simulink model "SAME5xPIM_MCLV2_MotorControl"  (R2020b)
settings: Solver=FixedStepDiscrete  StartTime=0.0  StopTime=10.0  FixedStep=0.0001  RelTol=1e-3  EnableMultiTasking=on
InitFcn:
  | % DC Voltage
  | VDC = 24;
  | 
  | % Intersective PMW
  | Vmax = VDC/2;
  | Imax = 4;
  | 
  | Ts = 1e-4;
  | 
  | 
  | % pole paires
  | p = 4;
  | 
  | % QEI
  | lines = 4*1000;
  | eleclines = lines/p;
  | inveleclines = 1/eleclines
  | gainQEIspeed = 2*pi/Ts/lines
  | 
  | % Electrical parameters
  | R=0.656; L=0.35e-3; Phif=0.0066;
  | % Mechanical parameters
  | F=1.e-05; J=1e-05; C0 = 0.01;%10;%1;
undefined symbols (not defined in the file or in its folder): ADC0, AIN0, DiscIntNeverNeededParam, PA02, PA03, PA08, PA09, PA10, PA11, PA12, PA13, PA16, PA17, PA18, pad0, pad1, pad2, pad3, PB08, PC16, PC17, PC18, Pin, SAME54P20A, TQFP128, VREFA, wo0, wo1, wo2, wo4, wo5, wo6
libraries: simulink x14, MCHP_Blockset x12, dsparch4 x1
(part 2 of 2)

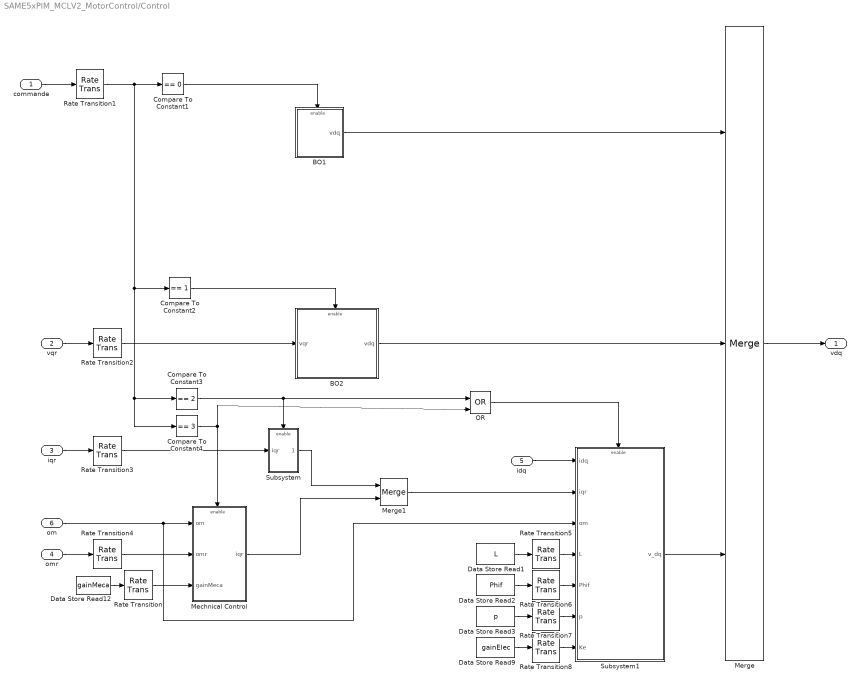
== system SAME5xPIM_MCLV2_MotorControl/Control ==
  commande : Inport
  vqr : Inport  Port=2
  iqr : Inport  Port=3
  omr : Inport  Port=4
  idq : Inport  Port=5
  om : Inport  Port=6
  BO1 : Subsystem
  BO2 : Subsystem
  Compare To Constant1 : simulink/Logic and Bit Operations/Compare To Constant  relop===  const=0  OutDataTypeStr=boolean
  Compare To Constant2 : simulink/Logic and Bit Operations/Compare To Constant  relop===  const=1  OutDataTypeStr=boolean
  Compare To Constant3 : simulink/Logic and Bit Operations/Compare To Constant  relop===  const=2  OutDataTypeStr=boolean
  Compare To Constant4 : simulink/Logic and Bit Operations/Compare To Constant  relop===  const=3  OutDataTypeStr=boolean
  Data Store Read1 : DataStoreRead  DataStoreName=L  SampleTime=1
  Data Store Read12 : DataStoreRead  DataStoreName=gainMeca  SampleTime=1
  Data Store Read2 : DataStoreRead  DataStoreName=Phif  SampleTime=1
  Data Store Read3 : DataStoreRead  DataStoreName=p  SampleTime=1
  Data Store Read9 : DataStoreRead  DataStoreName=gainElec  SampleTime=1
  Mechnical Control : Subsystem
  Merge : Merge  Inputs=3
  Merge1 : Merge
  OR : Logic  Operator=OR  IconShape=distinctive  AllPortsSameDT=off  OutDataTypeStr=boolean
  Rate Transition{,1..8} (9 alike) : RateTransition
  Subsystem : Subsystem
  Subsystem1 : Subsystem
  vdq : Outport  VectorParamsAs1DForOutWhenUnconnected=off
  wires:
  Rate Transition8/1 -> Subsystem1/7(Ke)
  Rate Transition7/1 -> Subsystem1/6(p)
  Rate Transition6/1 -> Subsystem1/5(Phif)
  Rate Transition5/1 -> Subsystem1/4(L)
  Rate Transition/1 -> Mechnical Control/3(gainMeca)
  Rate Transition4/1 -> Mechnical Control/2(omr)
  Rate Transition3/1 -> Subsystem/1(iqr)
  Rate Transition2/1 -> BO2/1(vqr)
  Subsystem1/1(v_dq) -> Merge/3
  Merge1/1 -> Subsystem1/2(iqr)
  idq/1 -> Subsystem1/1(idq)
  OR/1 -> Subsystem1/Enable
  om/1 -> Mechnical Control/1(om), Subsystem1/3(om)
  Compare To Constant4/1 -> Mechnical Control/Enable, OR/2
  Mechnical Control/1(iqr) -> Merge1/2
  Subsystem/1(Out1) -> Merge1/1
  Rate Transition1/1 -> Compare To Constant1/1, Compare To Constant4/1, Compare To Constant3/1, Compare To Constant2/1
  Compare To Constant3/1 -> Subsystem/Enable, OR/1
  Compare To Constant1/1 -> BO1/Enable
  commande/1 -> Rate Transition1/1
  Merge/1 -> vdq/1
  Compare To Constant2/1 -> BO2/Enable
  BO1/1(vdq) -> Merge/1
  BO2/1(vdq) -> Merge/2
  Data Store Read9/1 -> Rate Transition8/1
  Data Store Read1/1 -> Rate Transition5/1
  Data Store Read3/1 -> Rate Transition7/1
  Data Store Read2/1 -> Rate Transition6/1
  vqr/1 -> Rate Transition2/1
  iqr/1 -> Rate Transition3/1
  omr/1 -> Rate Transition4/1
  Data Store Read12/1 -> Rate Transition/1

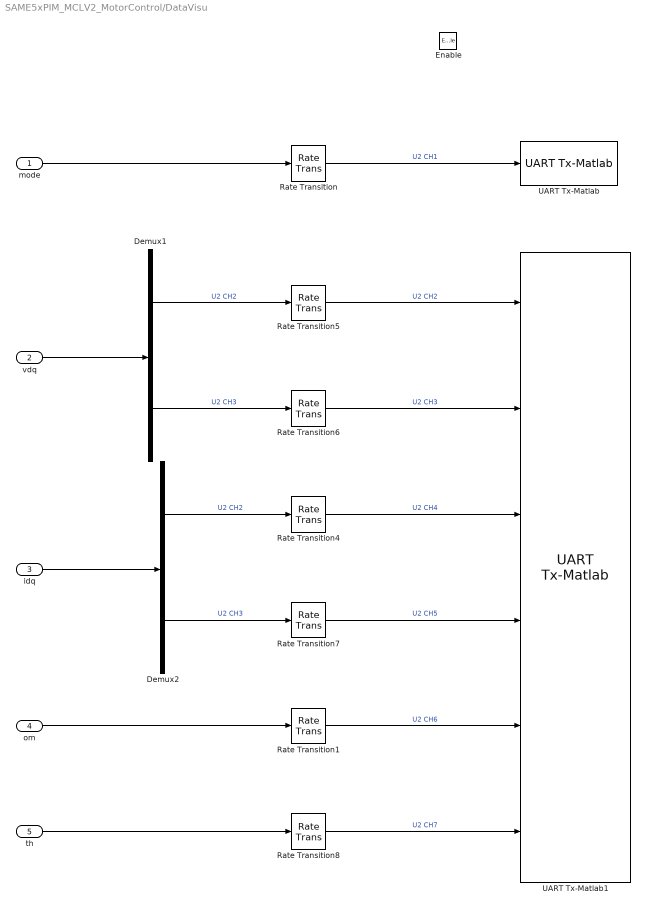
== system SAME5xPIM_MCLV2_MotorControl/DataVisu ==
  mode : Inport
  vdq : Inport  Port=2
  idq : Inport  Port=3
  om : Inport  Port=4
  th : Inport  Port=5
  Enable : EnablePort
  Demux1 : Demux  Outputs=2
  Demux2 : Demux  Outputs=2
  Rate Transition{,1,4..8} (7 alike) : RateTransition
  UART Tx-Matlab : MCHP_Blockset/BUS UART/UART Tx-Matlab  UART_REF=2  CHANNELS=[1]  AllOrNothing=off  SampleTime=.1  MCHP_MASTERLINK=SAME5xPIM_MCLV2_MotorControl/Microchip Master  MCHP_COMPILED_INFO="CompiledSampleTime= [0.10000000000000000555   0 ];CompiledInportDataTypes=[  5 ];CompiledInportDataWidth=[1];"
      settings: SourceProductName=MPLAB Device Blocks for Simulink
  UART Tx-Matlab1 : MCHP_Blockset/BUS UART/UART Tx-Matlab  UART_REF=2  CHANNELS=[2:7]  AllOrNothing=off  SampleTime=0.0005  MCHP_MASTERLINK=SAME5xPIM_MCLV2_MotorControl/Microchip Master  MCHP_COMPILED_INFO="CompiledSampleTime= [0.00050000000000000001041   0 ];CompiledInportDataTypes=[  1   1   1   1   1   1 ];CompiledInportDataWidth=[1  1  1  1  1  1];"
      settings: SourceProductName=MPLAB Device Blocks for Simulink
  wires:
  vdq/1 -> Demux1/1
  idq/1 -> Demux2/1
  th/1 -> Rate Transition8/1
  Demux2/2 -> Rate Transition7/1  "U2 CH3"
  Demux2/1 -> Rate Transition4/1  "U2 CH2"
  Rate Transition5/1 -> UART Tx-Matlab1/1  "U2 CH2"
  Rate Transition8/1 -> UART Tx-Matlab1/6  "U2 CH7"
  Rate Transition1/1 -> UART Tx-Matlab1/5  "U2 CH6"
  Demux1/2 -> Rate Transition6/1  "U2 CH3"
  Rate Transition6/1 -> UART Tx-Matlab1/2  "U2 CH3"
  Rate Transition4/1 -> UART Tx-Matlab1/3  "U2 CH4"
  Demux1/1 -> Rate Transition5/1  "U2 CH2"
  om/1 -> Rate Transition1/1
  Rate Transition7/1 -> UART Tx-Matlab1/4  "U2 CH5"
  Rate Transition/1 -> UART Tx-Matlab/1  "U2 CH1"
  mode/1 -> Rate Transition/1

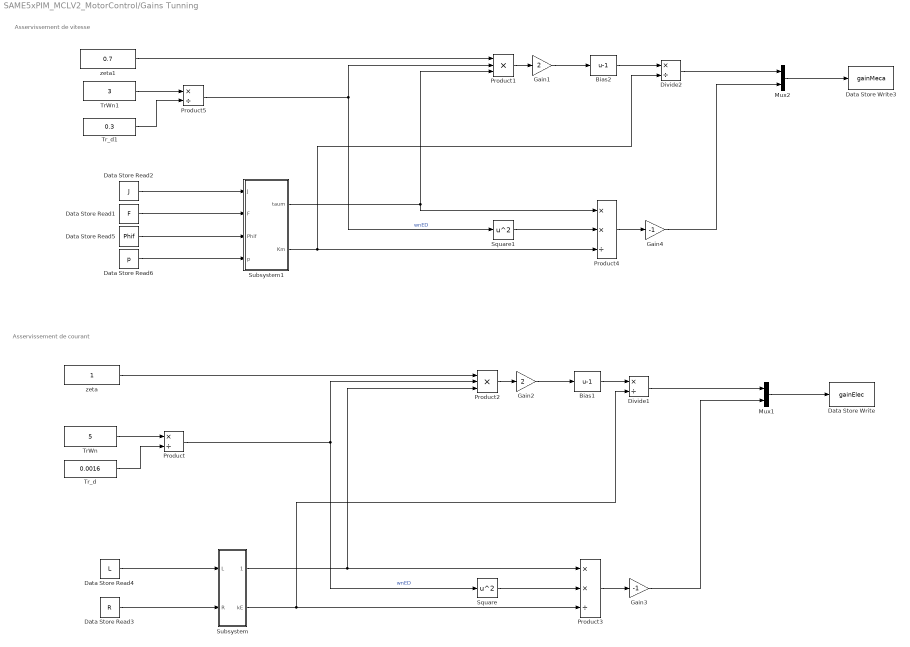
== system SAME5xPIM_MCLV2_MotorControl/Gains Tunning ==
  note: Asservissement de courant
  note: Asservissement de vitesse
  Bias1 : Bias  Bias=-1
  Bias2 : Bias  Bias=-1
  Data Store Read1 : DataStoreRead  DataStoreName=F  SampleTime=1
  Data Store Read2 : DataStoreRead  DataStoreName=J  SampleTime=1
  Data Store Read3 : DataStoreRead  DataStoreName=R  SampleTime=1
  Data Store Read4 : DataStoreRead  DataStoreName=L  SampleTime=1
  Data Store Read5 : DataStoreRead  DataStoreName=Phif  SampleTime=1
  Data Store Read6 : DataStoreRead  DataStoreName=p  SampleTime=1
  Data Store Write : DataStoreWrite  DataStoreName=gainElec  SampleTime=1
  Data Store Write3 : DataStoreWrite  DataStoreName=gainMeca
  Divide1 : Product  Inputs=*/
  Divide2 : Product  Inputs=*/
  Gain1 : Gain  Gain=2
  Gain2 : Gain  Gain=2
  Gain3 : Gain  Gain=-1
  Gain4 : Gain  Gain=-1
  Mux1 : Mux  Inputs=2
  Mux2 : Mux  Inputs=2
  Product : Product  Inputs=*/
  Product1 : Product  Inputs=3
  Product2 : Product  Inputs=3
  Product3 : Product  Inputs=**/
  Product4 : Product  Inputs=**/
  Product5 : Product  Inputs=*/
  Square : Math  Operator=square  SaturateOnIntegerOverflow=on
  Square1 : Math  Operator=square  SaturateOnIntegerOverflow=on
  Subsystem : Subsystem
  Subsystem1 : Subsystem
  TrWn : Constant  Value=5  OutDataTypeStr=single
  TrWn1 : Constant  Value=3  OutDataTypeStr=single
  Tr_d : Constant  Value=0.0016  OutDataTypeStr=single
  Tr_d1 : Constant  Value=0.3  OutDataTypeStr=single
  zeta : Constant  OutDataTypeStr=single
  zeta1 : Constant  Value=0.7  OutDataTypeStr=single
  wires:
  Gain3/1 -> Mux1/2
  Product3/1 -> Gain3/1
  Divide1/1 -> Mux1/1
  Bias1/1 -> Divide1/1
  Product2/1 -> Gain2/1
  Mux1/1 -> Data Store Write/1
  Data Store Read4/1 -> Subsystem/1(L)
  Data Store Read3/1 -> Subsystem/2(R)
  Subsystem/1(tauE) -> Product2/3, Product3/1
  TrWn/1 -> Product/1
  Tr_d/1 -> Product/2
  Product/1 -> Product2/2, Square/1  "wnED"
  Subsystem/2(kE) -> Divide1/2, Product3/3
  Gain2/1 -> Bias1/1
  zeta/1 -> Product2/1
  Square/1 -> Product3/2
  Square1/1 -> Product4/2
  Gain1/1 -> Bias2/1
  Product1/1 -> Gain1/1
  Bias2/1 -> Divide2/1
  Divide2/1 -> Mux2/1
  Product4/1 -> Gain4/1
  Gain4/1 -> Mux2/2
  Mux2/1 -> Data Store Write3/1
  Data Store Read2/1 -> Subsystem1/1(J)
  Data Store Read1/1 -> Subsystem1/2(F)
  Data Store Read5/1 -> Subsystem1/3(Phif)
  Data Store Read6/1 -> Subsystem1/4(p)
  Tr_d1/1 -> Product5/2
  TrWn1/1 -> Product5/1
  zeta1/1 -> Product1/1
  Product5/1 -> Square1/1, Product1/2  "wnED"
  Subsystem1/1(taum) -> Product4/1, Product1/3
  Subsystem1/2(Km) -> Divide2/2, Product4/3

== system SAME5xPIM_MCLV2_MotorControl/Inv Park ==
  cossin : Inport
  vdq : Inport  Port=2
  Clakeinv : Subsystem
  ParkInv : Subsystem
  vabc : Outport  VectorParamsAs1DForOutWhenUnconnected=off
  wires:
  vdq/1 -> ParkInv/2(vdq)
  cossin/1 -> ParkInv/1(cos(pth)sin(pth))
  ParkInv/1(valbe) -> Clakeinv/1(alphabeta)
  Clakeinv/1(abc) -> vabc/1

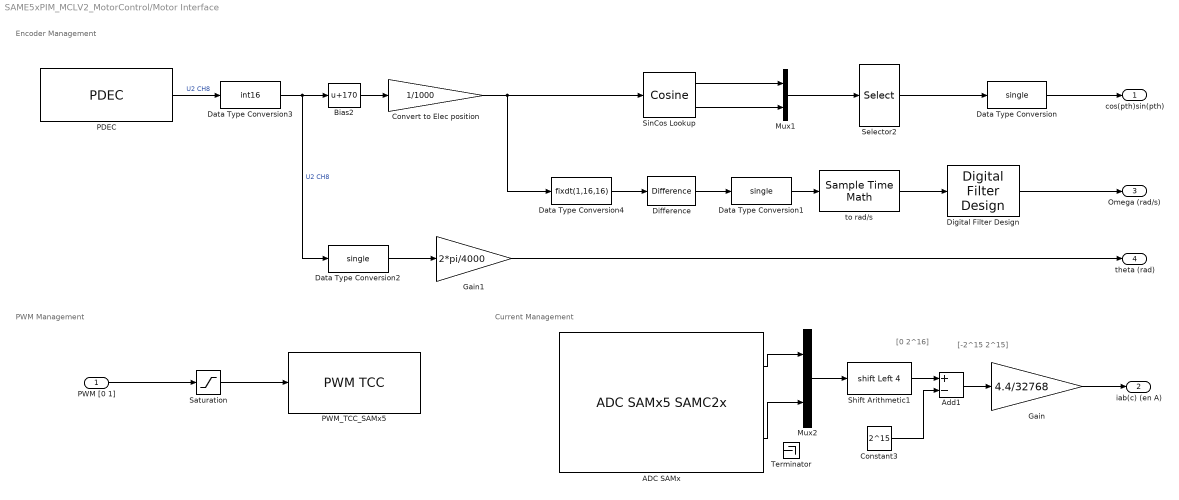
== system SAME5xPIM_MCLV2_MotorControl/Motor Interface ==
  note: [-2^15 2^15]
  note: [0 2^16]
  note: Encoder Management
  note: PWM Management
  note: Current Management
  PWM [0 1] : Inport
  ADC SAMx : MCHP_Blockset/Analog IO/ADC SAMx5 SAMC2x  ADCREF=ADC 0 and ADC 1 (slave)  VREF_seq0=Dynamic Options  VREF_seq0_TXT=PA03 / VREFA / Pin[10]  info=0  SampleTime=1e-4  MCHP_PORT={ADC0_seq0.0}{ADC0_AIN0}15:2:P2;{ADC1_seq0.0}{ADC1_AIN0}15:2:P40;  MCHP_MASTERLINK=SAME5xPIM_MCLV2_MotorControl/Microchip Master  MCHP_CRC=4658831  TrigSource_seq0=Dynamic Options  TrigSource_seq0_TXT=after this block evaluation  ADC0_seq0=Dynamic Options  ADC0_seq0_TXT=PA02 / AIN0 / Pin[9]  ADC1_seq0=Dynamic Options  ADC1_seq0_TXT=PB08 / AIN0 / Pin[19]  ADC0_seq0_1=Dynamic Options  ADC0_seq0_1_TXT=Not Used  ADC1_seq0_1=Dynamic Options  ADC1_seq0_1_TXT=Not Used  ADC0_seq0_2=Dynamic Options  ADC0_seq0_2_TXT=Not Used  ADC1_seq0_2=Dynamic Options  ADC1_seq0_2_TXT=Not Used  ADC0_seq0_3=Dynamic Options  ADC0_seq0_3_TXT=Not Used  ADC1_seq0_3=Dynamic Options  ADC1_seq0_3_TXT=Not Used  ADC0_seq0_4=Dynamic Options  ADC0_seq0_4_TXT=Not Used  ADC1_seq0_4=Dynamic Options  ADC1_seq0_4_TXT=Not Used  ADC0_seq0_5=Dynamic Options  ADC0_seq0_5_TXT=Not Used  ADC1_seq0_5=Dynamic Options  ADC1_seq0_5_TXT=Not Used  Resolution_seq0=12 bits  SampleTime_seq0_s=1e-6  TrigTimeStep_seq0=on  info_seq0=0  TrigSource_seq1=Dynamic Options  TrigSource_seq1_TXT=after this block evaluation  ADC0_seq1=Dynamic Options  ADC0_seq1_TXT=Not Used  ADC1_seq1=Dynamic Options  ADC1_seq1_TXT=Not Used  ADC0_seq1_1=Dynamic Options  ADC0_seq1_1_TXT=Not Used  ADC1_seq1_1=Dynamic Options  ADC1_seq1_1_TXT=Not Used  ADC0_seq1_2=Dynamic Options  ADC0_seq1_2_TXT=Not Used  ADC1_seq1_2=Dynamic Options  ADC1_seq1_2_TXT=Not Used  ADC0_seq1_3=Dynamic Options  ADC0_seq1_3_TXT=Not Used  ADC1_seq1_3=Dynamic Options  ADC1_seq1_3_TXT=Not Used  ADC0_seq1_4=Dynamic Options  ADC0_seq1_4_TXT=Not Used  ADC1_seq1_4=Dynamic Options  ADC1_seq1_4_TXT=Not Used  ADC0_seq1_5=Dynamic Options  ADC0_seq1_5_TXT=Not Used  ADC1_seq1_5=Dynamic Options  ADC1_seq1_5_TXT=Not Used  Resolution_seq1=12 bits  SampleTime_seq1_s=1e-6  TrigTimeStep_seq1=off  info_seq1=0  TrigSource_seq2=Dynamic Options  TrigSource_seq2_TXT=after this block evaluation  ADC0_seq2=Dynamic Options  ADC0_seq2_TXT=Not Used  ADC1_seq2=Dynamic Options  ADC1_seq2_TXT=Not Used  ADC0_seq2_1=Dynamic Options  ADC0_seq2_1_TXT=Not Used  ADC1_seq2_1=Dynamic Options  ADC1_seq2_1_TXT=Not Used  ADC0_seq2_2=Dynamic Options  ADC0_seq2_2_TXT=Not Used  ADC1_seq2_2=Dynamic Options  ADC1_seq2_2_TXT=Not Used  ADC0_seq2_3=Dynamic Options  ADC0_seq2_3_TXT=Not Used  ADC1_seq2_3=Dynamic Options  ADC1_seq2_3_TXT=Not Used  ADC0_seq2_4=Dynamic Options  ADC0_seq2_4_TXT=Not Used  ADC1_seq2_4=Dynamic Options  ADC1_seq2_4_TXT=Not Used  ADC0_seq2_5=Dynamic Options  ADC0_seq2_5_TXT=Not Used  ADC1_seq2_5=Dynamic Options  ADC1_seq2_5_TXT=Not Used  Resolution_seq2=12 bits  SampleTime_seq2_s=1e-6  TrigTimeStep_seq2=off  info_seq2=0  TrigSource_seq3=Dynamic Options  TrigSource_seq3_TXT=after this block evaluation  ADC0_seq3=Dynamic Options  ADC0_seq3_TXT=Not Used  ADC1_seq3=Dynamic Options  ADC1_seq3_TXT=Not Used  ADC0_seq3_1=Dynamic Options  ADC0_seq3_1_TXT=Not Used  ADC1_seq3_1=Dynamic Options  ADC1_seq3_1_TXT=Not Used  ADC0_seq3_2=Dynamic Options  ADC0_seq3_2_TXT=Not Used  ADC1_seq3_2=Dynamic Options  ADC1_seq3_2_TXT=Not Used  ADC0_seq3_3=Dynamic Options  ADC0_seq3_3_TXT=Not Used  ADC1_seq3_3=Dynamic Options  ADC1_seq3_3_TXT=Not Used  ADC0_seq3_4=Dynamic Options  ADC0_seq3_4_TXT=Not Used  ADC1_seq3_4=Dynamic Options  ADC1_seq3_4_TXT=Not Used  ADC0_seq3_5=Dynamic Options  ADC0_seq3_5_TXT=Not Used  ADC1_seq3_5=Dynamic Options  ADC1_seq3_5_TXT=Not Used  Resolution_seq3=12 bits  SampleTime_seq3_s=1e-6  TrigTimeStep_seq3=off  info_seq3=0  TrigSource_seq4=Dynamic Options  TrigSource_seq4_TXT=after this block evaluation  ADC0_seq4=Dynamic Options  ADC0_seq4_TXT=Not Used  ADC1_seq4=Dynamic Options  ADC1_seq4_TXT=Not Used  ADC0_seq4_1=Dynamic Options  ADC0_seq4_1_TXT=Not Used  ADC1_seq4_1=Dynamic Options  ADC1_seq4_1_TXT=Not Used  ADC0_seq4_2=Dynamic Options  ADC0_seq4_2_TXT=Not Used  ADC1_seq4_2=Dynamic Options  ADC1_seq4_2_TXT=Not Used  ADC0_seq4_3=Dynamic Options  ADC0_seq4_3_TXT=Not Used  ADC1_seq4_3=Dynamic Options  ADC1_seq4_3_TXT=Not Used  ADC0_seq4_4=Dynamic Options  ADC0_seq4_4_TXT=Not Used  ADC1_seq4_4=Dynamic Options  ADC1_seq4_4_TXT=Not Used  ADC0_seq4_5=Dynamic Options  ADC0_seq4_5_TXT=Not Used  ADC1_seq4_5=Dynamic Options  ADC1_seq4_5_TXT=Not Used  Resolution_seq4=12 bits  SampleTime_seq4_s=1e-6  TrigTimeStep_seq4=off  info_seq4=0  TrigSource_seq5=Dynamic Options  TrigSource_seq5_TXT=after this block evaluation  ADC0_seq5=Dynamic Options  ADC0_seq5_TXT=Not Used  ADC1_seq5=Dynamic Options  ADC1_seq5_TXT=Not Used  ADC0_seq5_1=Dynamic Options  ADC0_seq5_1_TXT=Not Used  ADC1_seq5_1=Dynamic Options  ADC1_seq5_1_TXT=Not Used  ADC0_seq5_2=Dynamic Options  ADC0_seq5_2_TXT=Not Used  ADC1_seq5_2=Dynamic Options  ADC1_seq5_2_TXT=Not Used  ADC0_seq5_3=Dynamic Options  ADC0_seq5_3_TXT=Not Used  ADC1_seq5_3=Dynamic Options  ADC1_seq5_3_TXT=Not Used  ADC0_seq5_4=Dynamic Options  ADC0_seq5_4_TXT=Not Used  ADC1_seq5_4=Dynamic Options  ADC1_seq5_4_TXT=Not Used  ADC0_seq5_5=Dynamic Options  ADC0_seq5_5_TXT=Not Used  ADC1_seq5_5=Dynamic Options  ADC1_seq5_5_TXT=Not Used  Resolution_seq5=12 bits  SampleTime_seq5_s=1e-6  TrigTimeStep_seq5=off  info_seq5=0
      settings: SourceProductName=MPLAB Device Blocks for Simulink
  Add1 : Sum  Inputs=+-  OutDataTypeStr=single
  Bias2 : Bias  Bias=170
  Constant3 : Constant  Value=2^15  OutDataTypeStr=fixdt(0,16,0)
  Convert to Elec position : Gain  Gain=1/1000  OutDataTypeStr=fixdt(0,16,16)
  Data Type Conversion : DataTypeConversion  OutDataTypeStr=single
  Data Type Conversion1 : DataTypeConversion  OutDataTypeStr=single
  Data Type Conversion2 : DataTypeConversion  OutDataTypeStr=single
  Data Type Conversion3 : DataTypeConversion  OutDataTypeStr=int16  ConvertRealWorld=Stored Integer (SI)
  Data Type Conversion4 : DataTypeConversion  OutDataTypeStr=fixdt(1,16,16)  ConvertRealWorld=Stored Integer (SI)
  Difference : simulink/Discrete/Difference  ICPrevInput=0  OutMin=[]  OutMax=[]  OutDataType=fixdt(1, 16)  OutScaling=2^-10  DoSatur=off
  Digital Filter Design : dsparch4/Digital Filter Design  mwdsp_browser_bugfix_var=off
  Gain : Gain  Gain=4.4/32768
  Gain1 : Gain  Gain=2*pi/4000
  Mux1 : Mux  Inputs=2
  Mux2 : Mux  Inputs=2
  PDEC : MCHP_Blockset/QEI/PDEC  Mode=Quadrature Encoder  index=Reset counter  QDI0=PC16 / Pin[70]  QDI0_txt=Dynamic Options  QDI1=PC17 / Pin[71]  QDI1_txt=Dynamic Options  QDI2=PC18 / Pin[72]  QDI2_txt=Dynamic Options  maxCounterReset=-1  AutoCorrection=off  AutoCorrection_override=on  info=0  MCHP_MASTERLINK=SAME5xPIM_MCLV2_MotorControl/Microchip Master  SampleTime=1e-4  MCHP_PORT={PDEC A}{PDEC_QDI0}5:0:P80;{PDEC B}{PDEC_QDI1}5:0:P81;{PDEC index}{PDEC_QDI2}5:0:P82;  MAXPOS_INPUT=off  RESET_INPUT=off  OutputCounter=on  OutputCounter_Signed=unsigned  OutputRevolution=off  CounterRevolution_length=Counter is 13 bits ; revolution is 3 bits  OutputRevolution_Signed=unsigned  FILTER="250 (ns)  ->  freq 2 (MHz)"  FILTER_TXT="250 (ns)  ->  freq 2 (MHz)"  SWAP=off  QDI_invert_0=off  QDI_invert_1=off  QDI_invert_2=off
      settings: SourceProductName=MPLAB Device Blocks for Simulink
  PWM_TCC_SAMx5 : MCHP_Blockset/PWM IO/PWM TCC  TCCREF=TCC 0  WAVE_choice=Center aligned PWM  MaxPeriod_s=5e-5  OTMX=Default  WO0=PA08 / Pin[33] / wo0  WO0_TXT=PA08 / Pin[33] / wo0  WO1=PA09 / Pin[34] / wo1  WO1_TXT=PA09 / Pin[34] / wo1  WO2=PA10 / Pin[35] / wo2  WO2_TXT=PA10 / Pin[35] / wo2  WO3=Not Used  WO3_TXT=Not Used  WO4=PA16 / Pin[66] / wo4  WO4_TXT=PA16 / Pin[66] / wo4  WO5=PA17 / Pin[67] / wo5  WO5_TXT=PA17 / Pin[67] / wo5  WO6=PA18 / Pin[68] / wo6  WO6_TXT=PA18 / Pin[68] / wo6  WO7=Not Used  WO7_TXT=Not Used  info=0  evalin_ws=PWM0max=MCHP_Fun.Hex2num('40A3860000000000');PWM0max=MCHP_Fun.Hex2num('40A3860000000000');PWM0max=MCHP_Fun.Hex2num('40A3860000000000');  SampleTime=1e-4  MCHP_PORT={PWM0_H0}{TCC0_WO0}5:1:P8;{PWM0_H1}{TCC0_WO1}5:1:P9;{PWM0_H2}{TCC0_WO2}5:1:P10;{PWM0_L0}{TCC0_WO4}5:1:P16;{PWM0_L1}{TCC0_WO5}5:1:P17;{PWM0_L2}{TCC0_WO6}5:1:P18;  MCHP_MASTERLINK=SAME5xPIM_MCLV2_MotorControl/Microchip Master  INVEN_WO0=off  INVEN_WO1=off  INVEN_WO2=off  INVEN_WO3=off  INVEN_WO4=off  INVEN_WO5=off  INVEN_WO6=off  INVEN_WO7=off  SWAP_PWM0=off  SWAP_PWM1=off  SWAP_PWM2=off  SWAP_PWM3=off  POL_PWM0=off  POL_PWM1=off  POL_PWM2=off  POL_PWM3=off  POL_PWM4=off  POL_PWM5=off  InitPeriod_s=5e-5  InitDutyCycle_s=2.5e-5  InitDeadTimeH_s=0.5e-6  InitDeadTimeL_s=0.5e-6  InitOutputOverride=0  InitOutputOverride_val=0  BlockInput_VectorScalar=Vectors (grouped by function)  BlockInput_Period=Not a block input  BlockInput_DutyCycle=a Floating Point input within range [0 1]  BlockInput_DeadTime=Not a block input  BlockInput_OutputOverride=Not a block input
      settings: SourceProductName=MPLAB Device Blocks for Simulink
  Saturation : Saturate  UpperLimit=0.98  LowerLimit=0.02  LinearizeAsGain=off  OutDataTypeStr=double
  Selector2 : Selector  InputPortWidth=2  IndexOptions=Index vector (dialog)  Indices=[2 1]  OutputSizes=1
  Shift Arithmetic1 : ArithShift  BitShiftNumber=4  BitShiftDirection=Left
  SinCos Lookup : simulink/Lookup Tables/Cosine  Formula=sin(2*pi*u) and cos(2*pi*u)  NumDataPoints=(2^12)+1  OutputWordLength=16  InternalRulePriority=Precision
      settings: SourceProductBaseCode=SL
  Terminator : Terminator
  to rad/s : SampleTimeMath  TsampMathOp=/  weightValue=4/(2*pi)
  cos(pth)sin(pth) : Outport  VectorParamsAs1DForOutWhenUnconnected=off
  iab(c) (en A) : Outport  Port=2  VectorParamsAs1DForOutWhenUnconnected=off
  Omega (rad/s) : Outport  Port=3  PortDimensions=1  VectorParamsAs1DForOutWhenUnconnected=off
  theta (rad) : Outport  Port=4  VectorParamsAs1DForOutWhenUnconnected=off
  wires:
  Saturation/1 -> PWM_TCC_SAMx5/1
  PWM [0 1]/1 -> Saturation/1
  ADC SAMx/1 -> Mux2/1
  ADC SAMx/2 -> Mux2/2
  Gain/1 -> iab(c) (en A)/1
  Shift Arithmetic1/1 -> Add1/1
  Mux2/1 -> Shift Arithmetic1/1
  Constant3/1 -> Add1/2
  Add1/1 -> Gain/1
  ? -> Terminator/1
  Data Type Conversion4/1 -> Difference/1
  Convert to Elec position/1 -> SinCos Lookup/1, Data Type Conversion4/1
  Data Type Conversion1/1 -> to rad/s/1
  to rad/s/1 -> Digital Filter Design/1
  Bias2/1 -> Convert to Elec position/1
  PDEC/1 -> Data Type Conversion3/1  "U2 CH8"
  Difference/1 -> Data Type Conversion1/1
  Digital Filter Design/1 -> Omega (rad/s)/1
  Data Type Conversion/1 -> cos(pth)sin(pth)/1
  Mux1/1 -> Selector2/1
  Selector2/1 -> Data Type Conversion/1
  SinCos Lookup/2 -> Mux1/2
  SinCos Lookup/1 -> Mux1/1
  Data Type Conversion3/1 -> Data Type Conversion2/1, Bias2/1  "U2 CH8"
  Data Type Conversion2/1 -> Gain1/1
  Gain1/1 -> theta (rad)/1

== system SAME5xPIM_MCLV2_MotorControl/PWM ==
  vabc : Inport
  50% average duty-cycle : Bias  Bias=0.5
  Gain : Gain  Gain=1/VDC  OutDataTypeStr=double
  PWM [0 1] : Outport  VectorParamsAs1DForOutWhenUnconnected=off
  wires:
  vabc/1 -> Gain/1
  50% average duty-cycle/1 -> PWM [0 1]/1
  Gain/1 -> 50% average duty-cycle/1

== system SAME5xPIM_MCLV2_MotorControl/Park  ==
  cossin : Inport
  xab(c) : Inport  Port=2
  Clark Fixe : Subsystem
  Park Fixe : Subsystem
  xdq : Outport  VectorParamsAs1DForOutWhenUnconnected=off
  wires:
  Clark Fixe/1(xalphabeta) -> Park Fixe/1(xalphabeta)
  xab(c)/1 -> Clark Fixe/1(xab(c))
  cossin/1 -> Park Fixe/2(cos(pth)sin(pth))
  Park Fixe/1(xdq) -> xdq/1

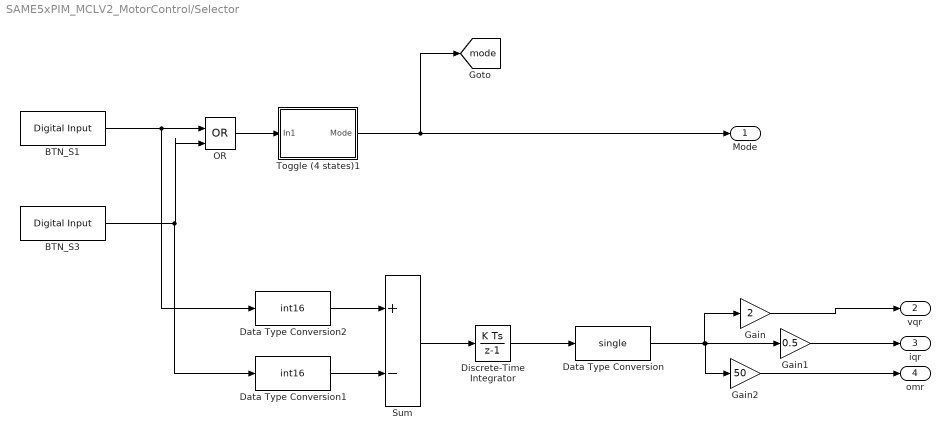
== system SAME5xPIM_MCLV2_MotorControl/Selector ==
  BTN_S1 : MCHP_Blockset/Digital IO/Digital Input  PORT=Dynamic Options  PORT_TXT="D   [ 0  1  8  9  10  11  12  20  21 ]"  PIN=9  PACK=off  SIMULTANEOUS=off  ORDERING=None  SampleTime=.1  MCHP_PORT={Digital In}{DIN}2:0:D9;  MCHP_MASTERLINK=SAME5xPIM_MCLV2_MotorControl/Microchip Master
      settings: SourceProductName=MPLAB Device Blocks for Simulink
  BTN_S3 : MCHP_Blockset/Digital IO/Digital Input  PORT=Dynamic Options  PORT_TXT="D   [ 0  1  8  9  10  11  12  20  21 ]"  PIN=10  PACK=off  SIMULTANEOUS=off  ORDERING=None  SampleTime=.1  MCHP_PORT={Digital In}{DIN}2:0:D10;  MCHP_MASTERLINK=SAME5xPIM_MCLV2_MotorControl/Microchip Master
      settings: SourceProductName=MPLAB Device Blocks for Simulink
  Data Type Conversion : DataTypeConversion  OutDataTypeStr=single
  Data Type Conversion1 : DataTypeConversion  OutDataTypeStr=int16
  Data Type Conversion2 : DataTypeConversion  OutDataTypeStr=int16
  Discrete-Time Integrator : DiscreteIntegrator  SampleTime=-1  LimitOutput=on  UpperSaturationLimit=7  LowerSaturationLimit=-7  ICPrevOutput=DiscIntNeverNeededParam  ICPrevScaledInput=DiscIntNeverNeededParam
  Gain : Gain  Gain=2
  Gain1 : Gain  Gain=0.5
  Gain2 : Gain  Gain=50
  OR : Logic  Operator=OR  IconShape=distinctive  AllPortsSameDT=off  OutDataTypeStr=boolean
  Sum : Sum  Inputs=+-
  Toggle (4 states)1 : Subsystem
  Mode : Outport  VectorParamsAs1DForOutWhenUnconnected=off
  vqr : Outport  Port=2  VectorParamsAs1DForOutWhenUnconnected=off
  iqr : Outport  Port=3  VectorParamsAs1DForOutWhenUnconnected=off
  omr : Outport  Port=4  VectorParamsAs1DForOutWhenUnconnected=off
  tag scope: mode=global
  wires:
  Discrete-Time Integrator/1 -> Data Type Conversion/1
  Sum/1 -> Discrete-Time Integrator/1
  Data Type Conversion1/1 -> Sum/2
  Data Type Conversion2/1 -> Sum/1
  OR/1 -> Toggle (4 states)1/1(In1)
  Gain2/1 -> omr/1
  Gain1/1 -> iqr/1
  Gain/1 -> vqr/1
  Data Type Conversion/1 -> Gain1/1, Gain2/1, Gain/1
  BTN_S3/1 -> OR/2, Data Type Conversion1/1
  Toggle (4 states)1/1(Mode) -> [mode], Mode/1
  BTN_S1/1 -> OR/1, Data Type Conversion2/1

== system SAME5xPIM_MCLV2_MotorControl/Control/BO1 ==
  Enable : EnablePort
  Mux : Mux  Inputs=2
  vd : Constant  Value=0  OutMin=[-12]  OutMax=[12]  OutDataTypeStr=single
  vq : Constant  Value=0  OutMin=[-12]  OutMax=[12]  OutDataTypeStr=single
  vdq : Outport  VectorParamsAs1DForOutWhenUnconnected=off
  wires:
  vd/1 -> Mux/1
  Mux/1 -> vdq/1
  vq/1 -> Mux/2

== system SAME5xPIM_MCLV2_MotorControl/Control/BO2 ==
  vqr : Inport
  Enable : EnablePort
  Constant : Constant  Value=0  OutDataTypeStr=single
  Mux : Mux  Inputs=2
  vdq : Outport  VectorParamsAs1DForOutWhenUnconnected=off
  wires:
  vqr/1 -> Mux/2
  Constant/1 -> Mux/1
  Mux/1 -> vdq/1

== system SAME5xPIM_MCLV2_MotorControl/Control/Mechnical Control ==
  om : Inport
  omr : Inport  Port=2
  gainMeca : Inport  Port=3
  Enable : EnablePort  StatesWhenEnabling=reset
  Augmented state feedback : Subsystem
      settings: PortSchema="{\"entries\":[{\"content\":{\"sides\":[{\"content\":{\"connectorIds\":[\"In1\",\"In2\"]},\"type\":\"ConnectorPlacement.EquallySpacedRectSide\",\"uuid\":\"89137e2f-cd18-4dcc-a524-9caf5367be1f\"},{\"content\":{\"connectorIds\":[\"Out1\"],\"side\":\"RIGHT\"},\"type\":\"ConnectorPlacement.EquallySpacedRectSide\",\"uuid\":\"4fa0fb61-d5d6-47b2-9e74-7b8a54a26f7d\"},{\"content\":{\"connectorIds\":[],\"side\":\"TOP\"},\"type\":\"ConnectorPlacement.EquallySpacedRectSide\",\"uuid\":\"143a26d0-3cb3-43f1-872c-87316c90bc9f\"},{\"content\":{\"connectorIds\":[\"In3\"],\"side\":\"BOTTOM\"},\"type\":\"ConnectorPlacement.EquallySpacedRectSide\",\"uuid\":\"8516086b-4f00-45b1-b860-126256ccf69b\"},{\"content\":{\"connectorIds\":[],\"side\":\"HIDDEN\"},\"type\":\"ConnectorPlacement.EquallySpacedRectSide\",\"uuid\":\"abbfb321-16c4-4def-9c9f-eddb440e6971\"}]},\"type\":\"ConnectorPlacement.EquallySpacedConnector\",\"uuid\":\"ad3527e6-0bb9-4e51-b689-1365c7b23b5d\"}],\"packageUris\":[\"http://schema.mathworks.com/mf0/Connector/R2020b\"],\"version\":\"1.0\"}"
  iqr : Outport  VectorParamsAs1DForOutWhenUnconnected=off
  wires:
  om/1 -> Augmented state feedback/2(om)
  Augmented state feedback/1(iqref) -> iqr/1
  omr/1 -> Augmented state feedback/1(omref)
  gainMeca/1 -> Augmented state feedback/3(gainMeca)

== system SAME5xPIM_MCLV2_MotorControl/Control/Subsystem ==
  iqr : Inport
  Enable : EnablePort
  Out1 : Outport
  wires:
  iqr/1 -> Out1/1

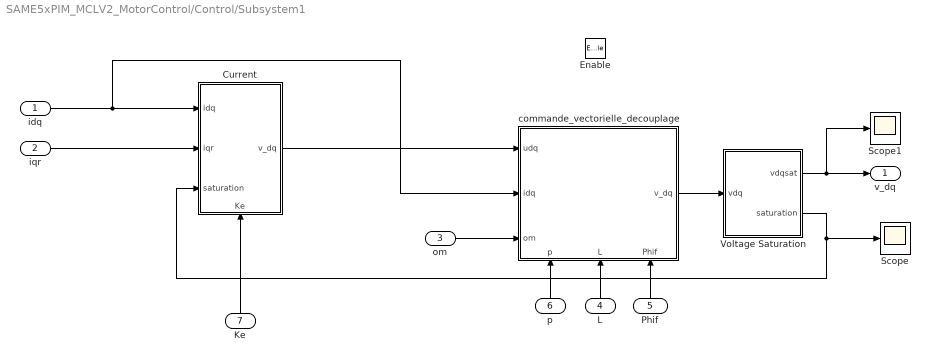
== system SAME5xPIM_MCLV2_MotorControl/Control/Subsystem1 ==
  idq : Inport
  iqr : Inport  Port=2
  om : Inport  Port=3
  L : Inport  Port=4
  Phif : Inport  Port=5
  p : Inport  Port=6
  Ke : Inport  Port=7
  Enable : EnablePort  StatesWhenEnabling=reset
  Current : Subsystem
      settings: PortSchema="{\"entries\":[{\"content\":{\"sides\":[{\"content\":{\"connectorIds\":[\"In1\",\"In2\",\"In3\"]},\"type\":\"ConnectorPlacement.EquallySpacedRectSide\",\"uuid\":\"0dd1bd5c-4f2d-4a51-9bc2-8bf74640d4ff\"},{\"content\":{\"connectorIds\":[\"Out1\"],\"side\":\"RIGHT\"},\"type\":\"ConnectorPlacement.EquallySpacedRectSide\",\"uuid\":\"9ff54608-efe8-47a2-97c0-1c2807ae0451\"},{\"content\":{\"connectorIds\":[],\"side\":\"TOP\"},\"type\":\"ConnectorPlacement.EquallySpacedRectSide\",\"uuid\":\"a5b0a1bc-2629-443b-a6ad-4c332df72e2c\"},{\"content\":{\"connectorIds\":[\"In4\"],\"side\":\"BOTTOM\"},\"type\":\"ConnectorPlacement.EquallySpacedRectSide\",\"uuid\":\"e8d63822-9705-4716-821c-9412f2966827\"},{\"content\":{\"connectorIds\":[],\"side\":\"HIDDEN\"},\"type\":\"ConnectorPlacement.EquallySpacedRectSide\",\"uuid\":\"63401b5c-75e9-49e9-aa08-12658d9987d3\"}]},\"type\":\"ConnectorPlacement.EquallySpacedConnector\",\"uuid\":\"d3f45542-3ea7-483a-a2ee-6c72d9ae8820\"}],\"packageUris\":[\"http://schema.mathworks.com/mf0/Connector/R2020b\"],\"version\":\"1.0\"}"
  Scope : Scope
  Scope1 : Scope
  Voltage Saturation : Subsystem
  commande_vectorielle_decouplage : Subsystem
      settings: PortSchema="{\"entries\":[{\"content\":{\"sides\":[{\"content\":{\"connectorIds\":[\"In1\",\"In2\",\"In3\"]},\"type\":\"ConnectorPlacement.EquallySpacedRectSide\",\"uuid\":\"169b5321-ee7c-423e-8449-192a786c9798\"},{\"content\":{\"connectorIds\":[\"Out1\"],\"side\":\"RIGHT\"},\"type\":\"ConnectorPlacement.EquallySpacedRectSide\",\"uuid\":\"910fdd05-0903-4759-8f85-a6669ffcf15d\"},{\"content\":{\"connectorIds\":[],\"side\":\"TOP\"},\"type\":\"ConnectorPlacement.EquallySpacedRectSide\",\"uuid\":\"8e0cf6ac-18cd-4e02-9312-1598b8dbe459\"},{\"content\":{\"connectorIds\":[\"In4\",\"In5\",\"In6\"],\"side\":\"BOTTOM\"},\"type\":\"ConnectorPlacement.EquallySpacedRectSide\",\"uuid\":\"bf7c0436-036d-4f64-97d8-e9b131650054\"},{\"content\":{\"connectorIds\":[],\"side\":\"HIDDEN\"},\"type\":\"ConnectorPlacement.EquallySpacedRectSide\",\"uuid\":\"cd87405f-25ee-425b-a181-6989070156fa\"}]},\"type\":\"ConnectorPlacement.EquallySpacedConnector\",\"uuid\":\"912b1b6f-c896-42c8-9325-248c15d73689\"}],\"packageUris\":[\"http://schema.mathworks.com/mf0/Connector/R2020b\"],\"version\":\"1.0\"}"
  v_dq : Outport
  wires:
  om/1 -> commande_vectorielle_decouplage/3(om)
  L/1 -> commande_vectorielle_decouplage/5(L)
  Phif/1 -> commande_vectorielle_decouplage/6(Phif)
  p/1 -> commande_vectorielle_decouplage/4(p)
  Voltage Saturation/1(vdqsat) -> Scope1/1, v_dq/1
  iqr/1 -> Current/2(iqr)
  Current/1(v_dq) -> commande_vectorielle_decouplage/1(udq)
  idq/1 -> commande_vectorielle_decouplage/2(idq), Current/1(idq)
  Ke/1 -> Current/4(Ke)
  Voltage Saturation/2(saturation) -> Scope/1, Current/3(saturation)
  commande_vectorielle_decouplage/1(v_dq) -> Voltage Saturation/1(vdq)

== system SAME5xPIM_MCLV2_MotorControl/Gains Tunning/Subsystem ==
  L : Inport
  R : Inport  Port=2
  Divide1 : Product  Inputs=/
  Divide2 : Product  Inputs=*/
  tauE : Outport
  kE : Outport  Port=2
  wires:
  Divide2/1 -> tauE/1  "tauE"
  R/1 -> Divide1/1, Divide2/2
  L/1 -> Divide2/1
  Divide1/1 -> kE/1  "kE"

== system SAME5xPIM_MCLV2_MotorControl/Gains Tunning/Subsystem1 ==
  J : Inport
  F : Inport  Port=2
  Phif : Inport  Port=3
  p : Inport  Port=4
  Divide3 : Product  Inputs=*/
  Divide6 : Product  Inputs=*/
  Divide7 : Product  Inputs=**
  Gain : Gain  Gain=3/2
  taum : Outport
  Km : Outport  Port=2
  wires:
  Gain/1 -> Divide7/1
  F/1 -> Divide3/2, Divide6/2
  J/1 -> Divide6/1
  p/1 -> Divide7/2
  Divide3/1 -> Km/1  "Km"
  Phif/1 -> Gain/1
  Divide6/1 -> taum/1  "taum"
  Divide7/1 -> Divide3/1  "Km"

== system SAME5xPIM_MCLV2_MotorControl/Inv Park/Clakeinv ==
  alphabeta : Inport
  Clarke1 : Product  Multiplication=Matrix(*)  RndMeth=Simplest  OutDataTypeStr=Inherit: Same as first input
  Constant Magnitude : Constant  Value=[1 0 ; -1/2 sqrt(3)/2 ;-1/2 -sqrt(3)/2]'  OutDataTypeStr=Inherit: Inherit via back propagation  SampleTime=-1
  Math Function : Math  Operator=transpose  SignedPower=on  SaturateOnIntegerOverflow=on
  abc : Outport  VectorParamsAs1DForOutWhenUnconnected=off
  wires:
  alphabeta/1 -> Math Function/1
  Constant Magnitude/1 -> Clarke1/2
  Math Function/1 -> Clarke1/1
  Clarke1/1 -> abc/1

== system SAME5xPIM_MCLV2_MotorControl/Inv Park/ParkInv ==
  cos(pth)sin(pth) : Inport
  vdq : Inport  Port=2
  Demux : Demux  Outputs=2
  Demux1 : Demux  Outputs=2
  Mux : Mux  Inputs=2
  Product{,1..3} (4 alike) : Product
  Sum : Sum  Inputs=|+-
  Sum1 : Sum  Inputs=|++
  valbe : Outport  VectorParamsAs1DForOutWhenUnconnected=off
  wires:
  vdq/1 -> Demux1/1
  cos(pth)sin(pth)/1 -> Demux/1
  Sum/1 -> Mux/1
  Demux1/1 -> Product2/1, Product/1
  Demux1/2 -> Product3/1, Product1/1
  Sum1/1 -> Mux/2
  Product1/1 -> Sum/2
  Product/1 -> Sum/1
  Demux/1 -> Product3/2, Product/2
  Demux/2 -> Product2/2, Product1/2
  Mux/1 -> valbe/1
  Product2/1 -> Sum1/1
  Product3/1 -> Sum1/2

== system SAME5xPIM_MCLV2_MotorControl/Park /Clark Fixe ==
  note: Input is a vector of 3 elements, 3rd element is not beeing used
  note: k = 2/3 : invariant Magnitude
  xab(c) : Inport
  Clarke1 : Product  Multiplication=Matrix(*)  OutDataTypeStr=single  RndMeth=Convergent  SaturateOnIntegerOverflow=on
  Constant Magnitude : Constant  Value=[1 0 ; 1/sqrt(3) 2/sqrt(3) ];  OutDataTypeStr=single
  xalphabeta : Outport  VectorParamsAs1DForOutWhenUnconnected=off
  wires:
  Clarke1/1 -> xalphabeta/1
  Constant Magnitude/1 -> Clarke1/1
  xab(c)/1 -> Clarke1/2

== system SAME5xPIM_MCLV2_MotorControl/Park /Park Fixe ==
  xalphabeta : Inport
  cos(pth)sin(pth) : Inport  Port=2
  Demux : Demux  Outputs=2
  Demux1 : Demux  Outputs=2
  Mux : Mux  Inputs=2
  Product{,1..3} (4 alike) : Product
  Sum : Sum  Inputs=|++  SaturateOnIntegerOverflow=on
  Sum1 : Sum  Inputs=|-+  SaturateOnIntegerOverflow=on
  xdq : Outport  VectorParamsAs1DForOutWhenUnconnected=off
  wires:
  cos(pth)sin(pth)/1 -> Demux1/1
  Product2/1 -> Sum1/2
  Product1/1 -> Sum1/1
  Demux1/2 -> Product3/2, Product1/2
  Demux1/1 -> Product2/2, Product/2
  Product/1 -> Sum/1
  Product3/1 -> Sum/2
  Sum1/1 -> Mux/2
  Demux/2 -> Product3/1, Product2/1
  Demux/1 -> Product1/1, Product/1
  Sum/1 -> Mux/1
  Mux/1 -> xdq/1
  xalphabeta/1 -> Demux/1

== system SAME5xPIM_MCLV2_MotorControl/Selector/Toggle (4 states)1 ==
  In1 : Inport
  Bitwise Operator : simulink/Logic and Bit Operations/Bitwise Operator  logicop=AND  UseBitMask=on  BitMask=3  BitMaskRealWorld=Stored Integer
  Change when button is pressed : simulink/Logic and Bit Operations/Detect Decrease  vinit=0.0  OutDataTypeStr=uint8
  Sum : Sum  AccumDataTypeStr=uint16  OutDataTypeStr=uint16
  Unit Delay : UnitDelay  SampleTime=-1  HasFrameUpgradeWarning=on
  Mode : Outport  VectorParamsAs1DForOutWhenUnconnected=off
  wires:
  Change when button is pressed/1 -> Sum/1
  Bitwise Operator/1 -> Mode/1, Unit Delay/1
  Unit Delay/1 -> Sum/2
  Sum/1 -> Bitwise Operator/1
  In1/1 -> Change when button is pressed/1

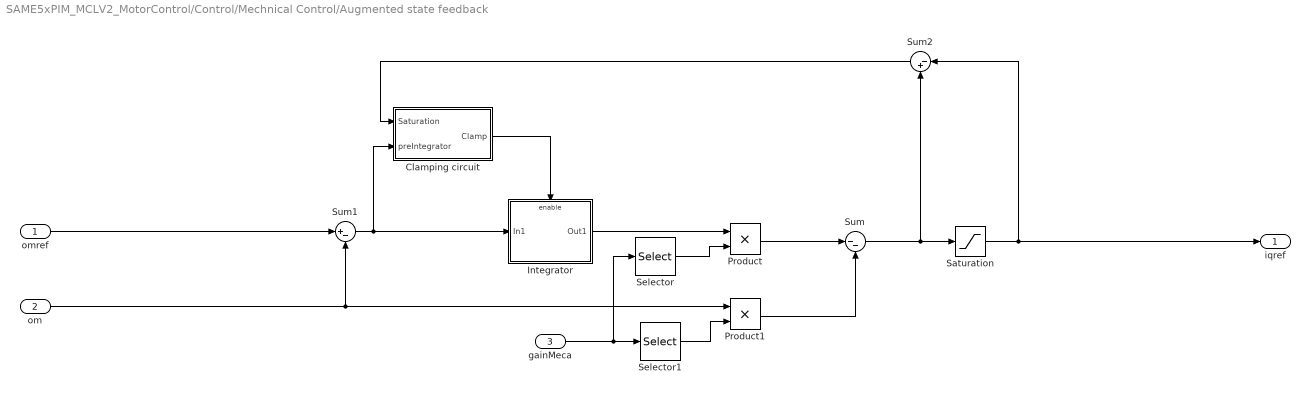
== system SAME5xPIM_MCLV2_MotorControl/Control/Mechnical Control/Augmented state feedback ==
  omref : Inport
  om : Inport  Port=2
  gainMeca : Inport  Port=3
  Clamping circuit : Subsystem
  Integrator : Subsystem
  Product : Product
  Product1 : Product
  Saturation : Saturate  UpperLimit=4  LowerLimit=-4
  Selector : Selector  InputPortWidth=2  IndexOptions=Index vector (dialog)  Indices=[2]  OutputSizes=1
  Selector1 : Selector  InputPortWidth=2  IndexOptions=Index vector (dialog)  Indices=1  OutputSizes=1
  Sum : Sum  Inputs=|--  OutDataTypeStr=single  SaturateOnIntegerOverflow=on
  Sum1 : Sum  Inputs=|+-
  Sum2 : Sum  Inputs=|-+  OutDataTypeStr=Inherit: Same as accumulator  SaturateOnIntegerOverflow=on
  iqref : Outport  VectorParamsAs1DForOutWhenUnconnected=off
  wires:
  Sum/1 -> Sum2/2, Saturation/1
  Product1/1 -> Sum/2
  Product/1 -> Sum/1
  om/1 -> Sum1/2, Product1/1
  Sum1/1 -> Integrator/1(In1), Clamping circuit/2(preIntegrator)
  omref/1 -> Sum1/1
  Clamping circuit/1(Clamp) -> Integrator/Enable
  Sum2/1 -> Clamping circuit/1(Saturation)
  Integrator/1(Out1) -> Product/1
  Saturation/1 -> Sum2/1, iqref/1
  Selector1/1 -> Product1/2
  Selector/1 -> Product/2
  gainMeca/1 -> Selector1/1, Selector/1

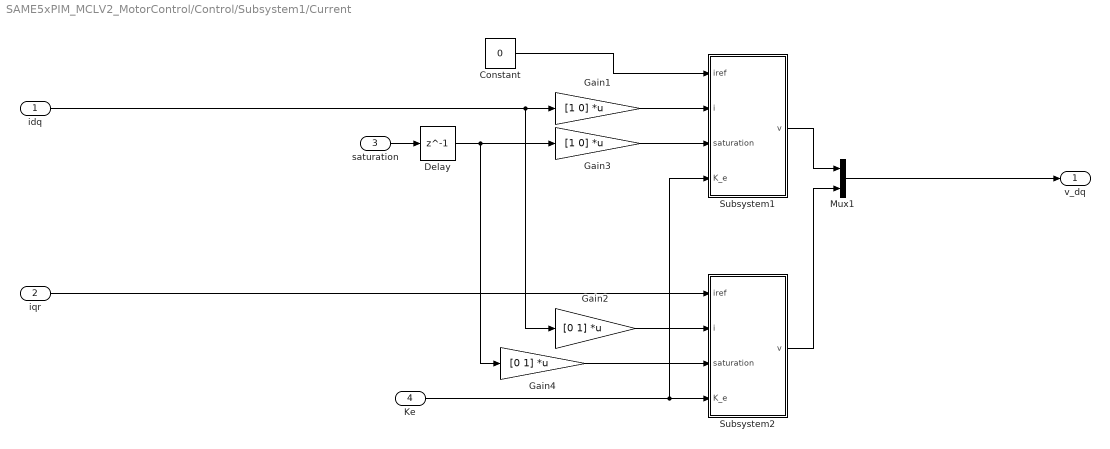
== system SAME5xPIM_MCLV2_MotorControl/Control/Subsystem1/Current ==
  idq : Inport
  iqr : Inport  Port=2
  saturation : Inport  Port=3
  Ke : Inport  Port=4
  Constant : Constant  Value=0
  Delay : Delay  DelayLength=1
  Gain1 : Gain  Gain=[1 0]  Multiplication=Matrix(K*u)  OutDataTypeStr=Inherit: Same as input
  Gain2 : Gain  Gain=[0 1]  Multiplication=Matrix(K*u)  OutDataTypeStr=Inherit: Same as input
  Gain3 : Gain  Gain=[1 0]  Multiplication=Matrix(K*u)  OutDataTypeStr=Inherit: Same as input
  Gain4 : Gain  Gain=[0 1]  Multiplication=Matrix(K*u)  OutDataTypeStr=Inherit: Same as input
  Mux1 : Mux  Inputs=2
  Subsystem1 : Subsystem
  Subsystem2 : Subsystem
  v_dq : Outport  VectorParamsAs1DForOutWhenUnconnected=off
  wires:
  Constant/1 -> Subsystem1/1(iref)
  saturation/1 -> Delay/1
  Subsystem2/1(v) -> Mux1/2
  Subsystem1/1(v) -> Mux1/1
  idq/1 -> Gain2/1, Gain1/1
  Gain1/1 -> Subsystem1/2(i)
  Gain2/1 -> Subsystem2/2(i)
  Mux1/1 -> v_dq/1
  Ke/1 -> Subsystem1/4(K_e), Subsystem2/4(K_e)
  Delay/1 -> Gain3/1, Gain4/1
  Gain3/1 -> Subsystem1/3(saturation)
  Gain4/1 -> Subsystem2/3(saturation)
  iqr/1 -> Subsystem2/1(iref)

== system SAME5xPIM_MCLV2_MotorControl/Control/Subsystem1/Voltage Saturation ==
  vdq : Inport
  Divide : Product  Inputs=*/
  Gain : Gain  Gain=Vmax
  Norm L2 : Subsystem
  Sum : Sum  Inputs=|+-
  Switch : Switch  Criteria=u2 > Threshold  Threshold=Vmax
  vdqsat : Outport  VectorParamsAs1DForOutWhenUnconnected=off
  saturation : Outport  Port=2  VectorParamsAs1DForOutWhenUnconnected=off
  wires:
  Sum/1 -> saturation/1
  vdq/1 -> Switch/3, Sum/1, Divide/1, Norm L2/1(In1)
  Switch/1 -> vdqsat/1, Sum/2
  Divide/1 -> Gain/1
  Norm L2/1(y) -> Switch/2, Divide/2
  Gain/1 -> Switch/1

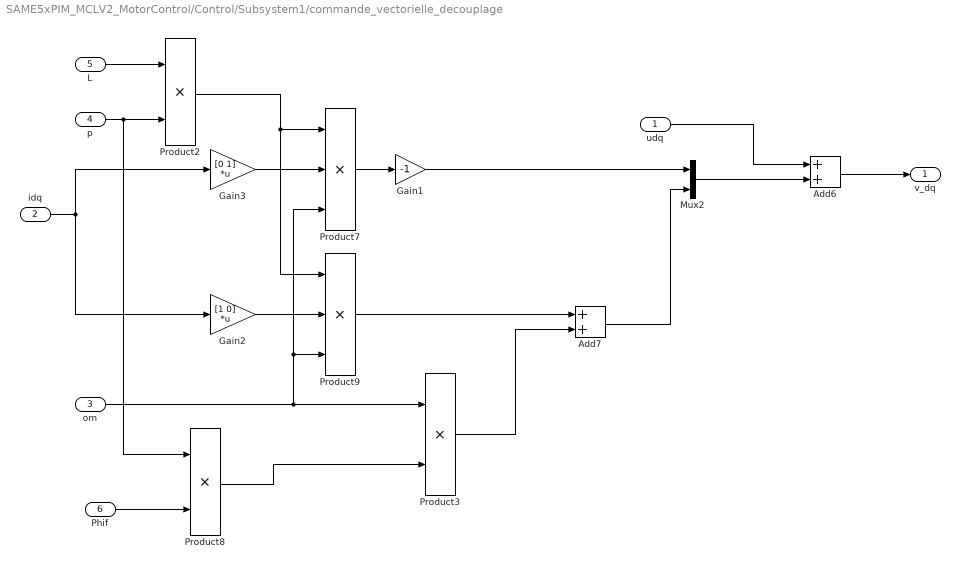
== system SAME5xPIM_MCLV2_MotorControl/Control/Subsystem1/commande_vectorielle_decouplage ==
  udq : Inport
  idq : Inport  Port=2
  om : Inport  Port=3
  p : Inport  Port=4
  L : Inport  Port=5
  Phif : Inport  Port=6
  Add6 : Sum
  Add7 : Sum
  Gain1 : Gain  Gain=-1
  Gain2 : Gain  Gain=[1 0]  Multiplication=Matrix(K*u)
  Gain3 : Gain  Gain=[0 1]  Multiplication=Matrix(K*u)
  Mux2 : Mux  Inputs=2
  Product2 : Product
  Product3 : Product
  Product7 : Product  Inputs=3
  Product8 : Product
  Product9 : Product  Inputs=3
  v_dq : Outport  VectorParamsAs1DForOutWhenUnconnected=off
  wires:
  Product3/1 -> Add7/2
  Product9/1 -> Add7/1
  Gain2/1 -> Product9/2
  om/1 -> Product7/3, Product9/3, Product3/1
  Product8/1 -> Product3/2
  Phif/1 -> Product8/2
  Product7/1 -> Gain1/1
  Gain3/1 -> Product7/2
  Product2/1 -> Product7/1, Product9/1
  L/1 -> Product2/1
  p/1 -> Product2/2, Product8/1
  Gain1/1 -> Mux2/1
  idq/1 -> Gain3/1, Gain2/1
  Add6/1 -> v_dq/1
  udq/1 -> Add6/1
  Add7/1 -> Mux2/2
  Mux2/1 -> Add6/2

== system SAME5xPIM_MCLV2_MotorControl/Control/Mechnical Control/Augmented state feedback/Clamping circuit ==
  note: The clamping enable or disable the integral action.
  Saturation : Inport  DisableCoverage=on
  preIntegrator : Inport  DisableCoverage=on  Port=2
  Compare To Zero1 : simulink/Logic and Bit Operations/Compare To Zero  relop=<=  OutDataTypeStr=boolean
  Delay : Delay  DelayLength=1  InitialCondition=0
  Multiply : Product
  Clamp : Outport  DisableCoverage=on  VectorParamsAs1DForOutWhenUnconnected=off
  wires:
  Delay/1 -> Multiply/1
  Saturation/1 -> Delay/1
  Multiply/1 -> Compare To Zero1/1
  preIntegrator/1 -> Multiply/2
  Compare To Zero1/1 -> Clamp/1

== system SAME5xPIM_MCLV2_MotorControl/Control/Mechnical Control/Augmented state feedback/Integrator ==
  In1 : Inport
  Enable : EnablePort
  Discrete-Time Integrator : DiscreteIntegrator  SampleTime=1e-4  OutDataTypeStr=single  SaturateOnIntegerOverflow=on  ICPrevOutput=DiscIntNeverNeededParam  ICPrevScaledInput=DiscIntNeverNeededParam
  Out1 : Outport  VectorParamsAs1DForOutWhenUnconnected=off
  wires:
  In1/1 -> Discrete-Time Integrator/1
  Discrete-Time Integrator/1 -> Out1/1

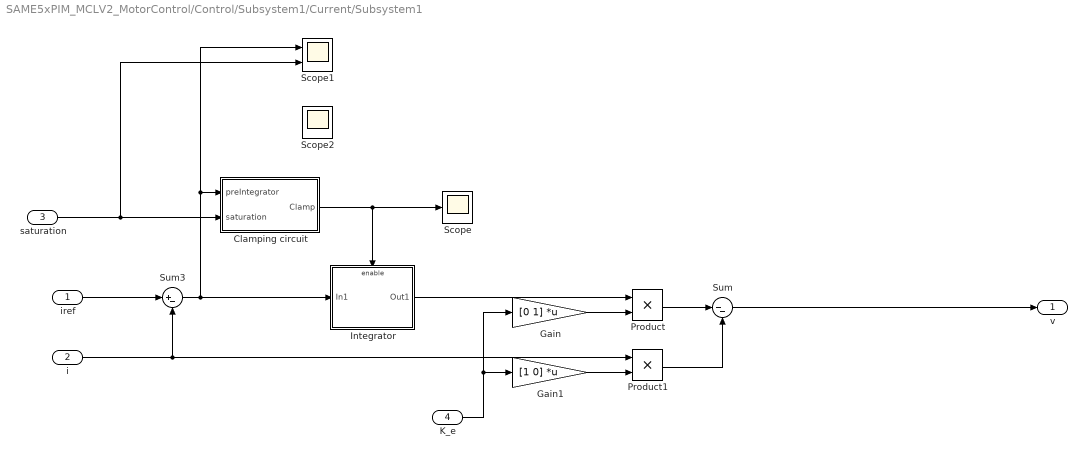
== system SAME5xPIM_MCLV2_MotorControl/Control/Subsystem1/Current/Subsystem1 ==
  iref : Inport
  i : Inport  Port=2
  saturation : Inport  Port=3
  K_e : Inport  Port=4
  Clamping circuit : Subsystem
  Gain : Gain  Gain=[0 1]  Multiplication=Matrix(K*u)
  Gain1 : Gain  Gain=[1 0]  Multiplication=Matrix(K*u)
  Integrator : Subsystem
  Product : Product
  Product1 : Product
  Scope : Scope
  Scope1 : Scope  NumInputPorts=2
  Scope2 : Scope
  Sum : Sum  Inputs=|--  OutDataTypeStr=single  SaturateOnIntegerOverflow=on
  Sum3 : Sum  Inputs=|+-
  v : Outport  VectorParamsAs1DForOutWhenUnconnected=off
  wires:
  Sum/1 -> v/1
  Integrator/1(Out1) -> Product/1
  Clamping circuit/1(Clamp) -> Scope/1, Integrator/Enable
  iref/1 -> Sum3/1
  Sum3/1 -> Integrator/1(In1), Scope1/1, Clamping circuit/1(preIntegrator)
  i/1 -> Sum3/2, Product1/1
  Product/1 -> Sum/1
  Product1/1 -> Sum/2
  K_e/1 -> Gain/1, Gain1/1
  Gain/1 -> Product/2
  Gain1/1 -> Product1/2
  saturation/1 -> Scope1/2, Clamping circuit/2(saturation)

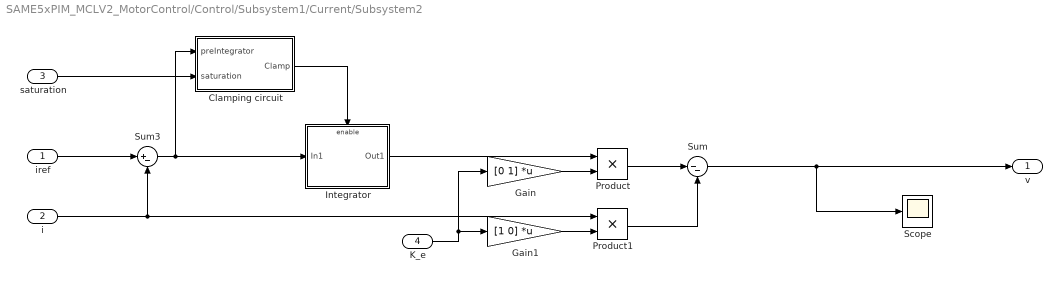
== system SAME5xPIM_MCLV2_MotorControl/Control/Subsystem1/Current/Subsystem2 ==
  iref : Inport
  i : Inport  Port=2
  saturation : Inport  Port=3
  K_e : Inport  Port=4
  Clamping circuit : Subsystem
  Gain : Gain  Gain=[0 1]  Multiplication=Matrix(K*u)
  Gain1 : Gain  Gain=[1 0]  Multiplication=Matrix(K*u)
  Integrator : Subsystem
  Product : Product
  Product1 : Product
  Scope : Scope
  Sum : Sum  Inputs=|--  OutDataTypeStr=single  SaturateOnIntegerOverflow=on
  Sum3 : Sum  Inputs=|+-
  v : Outport  VectorParamsAs1DForOutWhenUnconnected=off
  wires:
  saturation/1 -> Clamping circuit/2(saturation)
  Gain1/1 -> Product1/2
  Gain/1 -> Product/2
  K_e/1 -> Gain1/1, Gain/1
  Product1/1 -> Sum/2
  Product/1 -> Sum/1
  i/1 -> Product1/1, Sum3/2
  Sum3/1 -> Clamping circuit/1(preIntegrator), Integrator/1(In1)
  iref/1 -> Sum3/1
  Clamping circuit/1(Clamp) -> Integrator/Enable
  Integrator/1(Out1) -> Product/1
  Sum/1 -> Scope/1, v/1

== system SAME5xPIM_MCLV2_MotorControl/Control/Subsystem1/Voltage Saturation/Norm L2 ==
  In1 : Inport
  Dot Product : DotProduct  InputSameDT=on  OutDataTypeStr=Inherit: Inherit via internal rule
  Sqrt : Sqrt  SaturateOnIntegerOverflow=on
  y : Outport
  wires:
  In1/1 -> Dot Product/1, Dot Product/2
  Dot Product/1 -> Sqrt/1
  Sqrt/1 -> y/1

== system SAME5xPIM_MCLV2_MotorControl/Control/Subsystem1/Current/Subsystem1/Clamping circuit ==
  note: The clamping enable or disable the integral action.
  preIntegrator : Inport  DisableCoverage=on
  saturation : Inport  DisableCoverage=on  Port=2
  Compare To Zero1 : simulink/Logic and Bit Operations/Compare To Zero  relop=<=  OutDataTypeStr=boolean
  Multiply : Product
  Clamp : Outport  DisableCoverage=on  VectorParamsAs1DForOutWhenUnconnected=off
  wires:
  saturation/1 -> Multiply/1
  Compare To Zero1/1 -> Clamp/1
  Multiply/1 -> Compare To Zero1/1
  preIntegrator/1 -> Multiply/2

== system SAME5xPIM_MCLV2_MotorControl/Control/Subsystem1/Current/Subsystem1/Integrator ==
  In1 : Inport
  Enable : EnablePort
  Discrete-Time Integrator : DiscreteIntegrator  SampleTime=Ts  OutDataTypeStr=single  ICPrevOutput=DiscIntNeverNeededParam  ICPrevScaledInput=DiscIntNeverNeededParam
  Out1 : Outport  VectorParamsAs1DForOutWhenUnconnected=off
  wires:
  Discrete-Time Integrator/1 -> Out1/1
  In1/1 -> Discrete-Time Integrator/1

== system SAME5xPIM_MCLV2_MotorControl/Control/Subsystem1/Current/Subsystem2/Clamping circuit ==
  note: The clamping enable or disable the integral action.
  preIntegrator : Inport  DisableCoverage=on
  saturation : Inport  DisableCoverage=on  Port=2
  Compare To Zero1 : simulink/Logic and Bit Operations/Compare To Zero  relop=<=  OutDataTypeStr=boolean
  Multiply : Product
  Clamp : Outport  DisableCoverage=on  VectorParamsAs1DForOutWhenUnconnected=off
  wires:
  preIntegrator/1 -> Multiply/2
  Multiply/1 -> Compare To Zero1/1
  Compare To Zero1/1 -> Clamp/1
  saturation/1 -> Multiply/1

== system SAME5xPIM_MCLV2_MotorControl/Control/Subsystem1/Current/Subsystem2/Integrator ==
  In1 : Inport
  Enable : EnablePort
  Discrete-Time Integrator : DiscreteIntegrator  SampleTime=Ts  OutDataTypeStr=single  ICPrevOutput=DiscIntNeverNeededParam  ICPrevScaledInput=DiscIntNeverNeededParam
  Out1 : Outport  VectorParamsAs1DForOutWhenUnconnected=off
  wires:
  In1/1 -> Discrete-Time Integrator/1
  Discrete-Time Integrator/1 -> Out1/1
